simulink model "jidai"  (Simulink 6.0)
settings: Solver=ode45  StartTime=0.0  StopTime=10.0  RelTol=1e-3
undefined symbols (not defined in the file): rcosine
libraries: simulink x6, commsink2 x2, commrandsrc2 x1, dspswit3 x1, dsparch4 x1, commsynccomp2 x1, commutil2 x1, dspsigops x1
settings Model: LastModifiedBy=xxgcxy602

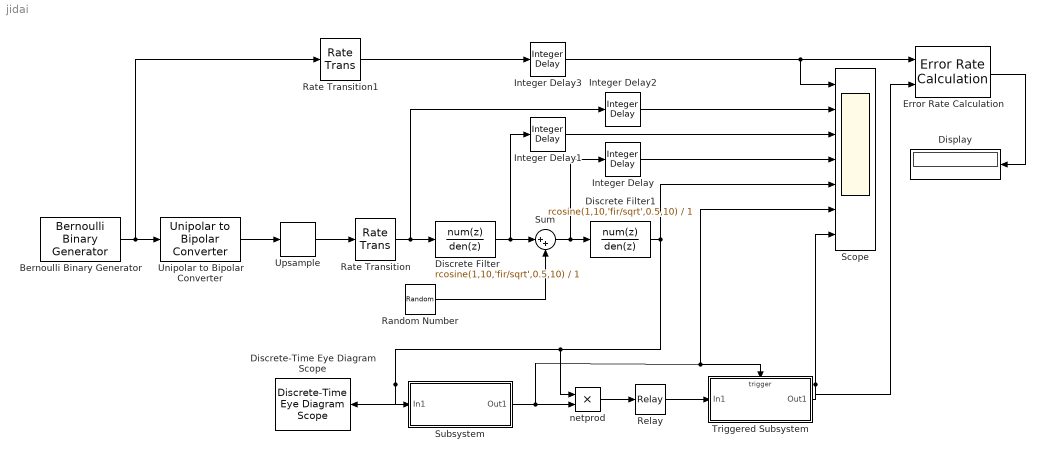
== system jidai ==
  Bernoulli Binary Generator : commrandsrc2/Bernoulli Binary Generator  P=0.5  seed=61  Ts=1/1000  frameBased=off  sampPerFrame=1  orient=off
  Discrete Filter : DiscreteFilter  Numerator=rcosine(1,10,'fir/sqrt',0.5,10)  Denominator=1
  Discrete Filter1 : DiscreteFilter  Numerator=rcosine(1,10,'fir/sqrt',0.5,10)  Denominator=1
  Discrete-Time Eye Diagram Scope : commsink2/Discrete-Time Eye Diagram Scope  Tag=EyeDiagram  Orientation=left  sampPerSymb=8  offsetEye=0  symbPerTrace=1  numTraces=40  numNewFrames=10  LineStyles=-  LineColors=b  dupPoints=on  fading=on  render=on  AxisGrid=on  yMin=-1.5  yMax=1.5  inphaseLabel=In-phase Amplitude  quadratureLabel=Quadrature Amplitude  openScopeAtSimStart=on  dispDiagram=In-phase and Quadrature  FrameNumber=off  FigPos=[403 24 560 644]  figTitle=Eye Diagram  block_type_=eye  numLinesMax=8
  Display : Display
  Error Rate Calculation : commsink2/Error Rate Calculation  N=0  st_delay=0  cp_mode=Entire frame  subframe=[]  PMode=Port  WsName=ErrorVec  RsMode2=off  stop=off  numErr=100  maxBits=1e6
  Integer Delay : simulink/Discrete/Integer Delay  vinit=0.0  samptime=-1  NumDelays=100
  Integer Delay1 : simulink/Discrete/Integer Delay  vinit=0.0  samptime=-1  NumDelays=100
  Integer Delay2 : simulink/Discrete/Integer Delay  vinit=0.0  samptime=-1  NumDelays=202
  Integer Delay3 : simulink/Discrete/Integer Delay  vinit=0.0  samptime=-1  NumDelays=207
  Random Number : RandomNumber  SampleTime=1/1000
  Rate Transition : RateTransition
  Rate Transition1 : RateTransition
  Relay : Relay  OnSwitchValue=0  OffSwitchValue=0
  Scope : Scope  NumInputPorts=7
      settings: YMin=-5~-5~-1~-2~-2~-5~-5  YMax=5~5~1~2~2~5~5
  Subsystem : Subsystem
  Sum : Sum  Inputs=|++
  Triggered Subsystem : Subsystem  TreatAsAtomicUnit=on
  Unipolar to Bipolar Converter : commutil2/Unipolar to Bipolar Converter  M=2  polarity=Positive
  Upsample : dspsigops/Upsample  N=2  phase=0  ic=0  mode=Maintain input frame size
  netprod : Product  SaturateOnIntegerOverflow=on  RndMeth=Zero  InputSameDT=on
  wires:
  Bernoulli Binary Generator/1 -> Unipolar to Bipolar Converter/1, Rate Transition1/1
  Unipolar to Bipolar Converter/1 -> Upsample/1
  Upsample/1 -> Rate Transition/1
  Rate Transition/1 -> Discrete Filter/1, Integer Delay2/1
  Discrete Filter/1 -> Sum/1, Integer Delay1/1
  Sum/1 -> Discrete Filter1/1, Integer Delay/1
  Rate Transition1/1 -> Integer Delay3/1
  Discrete Filter1/1 -> Scope/5, Subsystem/1(In1), Discrete-Time Eye Diagram Scope/1, netprod/1
  Integer Delay/1 -> Scope/4
  Integer Delay1/1 -> Scope/3
  Integer Delay2/1 -> Scope/2
  Random Number/1 -> Sum/2
  netprod/1 -> Relay/1
  Integer Delay3/1 -> Error Rate Calculation/1, Scope/1
  Error Rate Calculation/1 -> Display/1
  Subsystem/1(Out1) -> netprod/2, Triggered Subsystem/Trigger, Scope/6
  Relay/1 -> Triggered Subsystem/1(In1)
  Triggered Subsystem/1(Out1) -> Scope/7, Error Rate Calculation/2

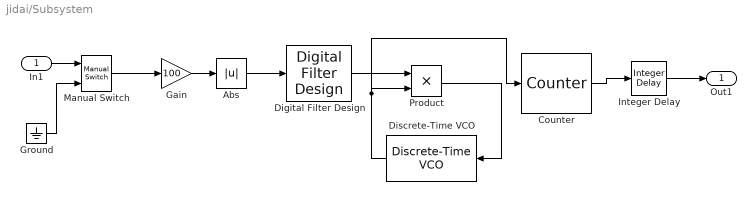
== system jidai/Subsystem ==
  In1 : Inport  Port=1  LatchInput=off
  Abs : Abs
  Counter : dspswit3/Counter  Direction=Up  CountEvent=Rising edge  CounterSize=User defined  MaxCount=1  InitialCount=0  Output=Count  HitValue=32  ResetInput=off  SamplesPerFrame=1  Ts=1  CntDtype=double  HitDtype=Logical
  Digital Filter Design : dsparch4/Digital Filter Design
  Discrete-Time VCO : commsynccomp2/Discrete-Time VCO  Orientation=left  Ac=1  Fc=1994  Kc=8  Ph=0  ts=1/10000
  Gain : Gain  Gain=100
  Ground : Ground
  Integer Delay : simulink/Discrete/Integer Delay  vinit=0.0  samptime=-1  NumDelays=4
  Manual Switch : simulink/Signal Routing/Manual Switch  sw=1  action=0
  Product : Product  RndMeth=Zero
  Out1 : Outport
  wires:
  Manual Switch/1 -> Gain/1
  In1/1 -> Manual Switch/1
  Ground/1 -> Manual Switch/2
  Gain/1 -> Abs/1
  Abs/1 -> Digital Filter Design/1
  Digital Filter Design/1 -> Product/1
  Discrete-Time VCO/1 -> Product/2, Counter/1
  Product/1 -> Discrete-Time VCO/1
  Integer Delay/1 -> Out1/1
  Counter/1 -> Integer Delay/1

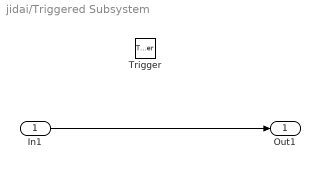
== system jidai/Triggered Subsystem ==
  In1 : Inport  Port=1  LatchInput=off
  Trigger : TriggerPort
  Out1 : Outport
  wires:
  In1/1 -> Out1/1
